simulink model "model"  (R2021a)
settings: Solver=VariableStepAuto  StartTime=0.0  StopTime=1.5  RelTol=1e-3
libraries: simulink x1
settings Model: Creator=alamg  LastModifiedBy=alamg

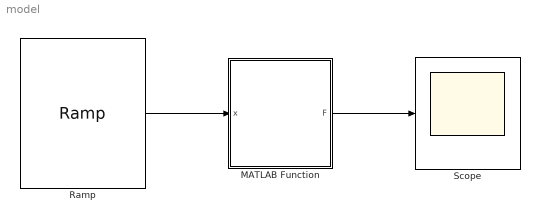
== system model ==
  MATLAB Function : MATLAB Function  TreatAsAtomicUnit=on
  Ramp : simulink/Sources/Ramp  slope=1  start=0  InitialOutput=0
  Scope : Scope
  wires:
  MATLAB Function/1(F) -> Scope/1
  Ramp/1 -> MATLAB Function/1(x)

== matlab function model/MATLAB Function ==
  data: x input; F output
function F = fcn(x)
b = sqrt(1+x^2);
F = 0.4/b - b*(1 - 0.4/b^2 )+x;
